simulink model "Lab_1.1_1.3"  (R2025a)
settings: Solver=FixedStepAuto  StartTime=0.0  StopTime=inf  RelTol=1e-3  EnableMultiTasking=on
libraries: fl_lib x18, nesl_utility x18, stm32f4xxblockslib x8, ee_lib x6, dspstat3 x2
settings Model: STM32="{\"AnalogInput\":[{\"ID\":\"test_poten:20\"},{\"ID\":\"test_poten:28\"},{\"ID\":\"ADC_reader:28\"},{\"ID\":\"ADC_reader:20\"},{\"ID\":\"ADC_reader:14\"},{\"ID\":\"ADC_reader:11\"},{\"ID\":\"ADC_reader:8\"},{\"ID\":\"ADC_reader:5\"},{\"ID\":\"ADC_reader:1\"},{\"ID\":\"ADC_reader_simulink:14\"},{\"ID\":\"ADC_reader_simulink:11\"},{\"ID\":\"ADC_reader_simulink:8\"},{\"ID\":\"ADC_reader_simulink:5\"},{\"ID\":\"ADC_reader_simulink:1\"},{\"ID\":\"ADC_reader_simulink:124\"},{\"ID\":\"ADC_reader_simulink:20\"}]}"  Creator=ioonz  LastModifiedBy=Ben
settings OptimizationCC: DefaultParameterBehavior=Inlined  EnhancedBackFolding=on  PassReuseOutputArgsAs=Individual arguments  ZeroExternalMemoryAtStartup=off  ZeroInternalMemoryAtStartup=off  MaxStackSize=512  OptimizeBlockOrder=speed  DifferentSizesBufferReuse=on  OptimizationCustomize=off  EfficientTunableParamExpr=on
settings DebuggingCC: ParameterTunabilityLossMsg=error
settings HardwareCC: ProdBitPerPointer=32.0  ProdBitPerSizeT=32.0  ProdBitPerPtrDiffT=32.0  ProdLargestAtomicInteger=Long  ProdLargestAtomicFloat=Double  ProdWordSize=32.0  ProdLongLongMode=on  ProdHWDeviceType=ARM Compatible->ARM Cortex-M
settings SFSimCC: MATLABDynamicMemAlloc=off
settings RTWCC: SystemTargetFile=ert.tlc  HardwareBoard=STM32G4xx Based  TemplateMakefile=ert_default_tmf  Toolchain=GNU Tools for ARM Embedded Processors  Description=Embedded Coder
settings CodeAppCC: ForceParamTrailComments=on  IgnoreCustomStorageClasses=off  OperatorAnnotations=on  SimulinkDataObjDesc=on  SFDataObjDesc=on  InsertBlockDesc=on
settings ERTTargetCC: ExtModeTransport=3.0  ExtModeStaticAllocSize=2048.0  TargetLangStandard=C99 (ISO)  CodeReplacementLibrary=ARM Cortex-M

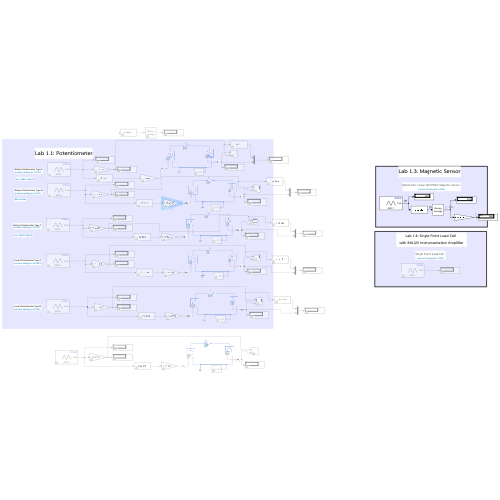
[thumbnail: Simulink's stored preview of the top-level diagram]
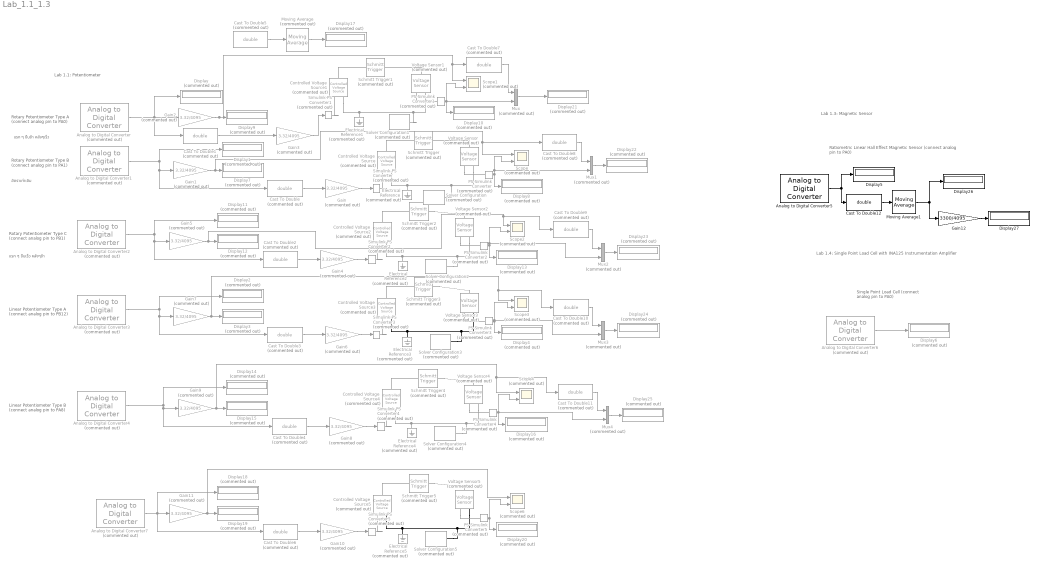
== system Lab_1.1_1.3 ==
  note: Lab 1.1: Potentiometer
  note: Rotary Potentiometer Type A
      | (connect analog pin to PA0)
  note: Rotary Potentiometer Type B
      | (connect analog pin to PA1)
  note: Rotary Potentiometer Type C
      | (connect analog pin to PB1)
  note: Linear Potentiometer Type A
      | (connect analog pin to PB12)
  note: Linear Potentiometer Type B
      | (connect analog pin to PA8)
  note: Ratiometric Linear Hall Effect Magnetic Sensor
      | (connect analog pin to PA0)
  note: Single Point Load Cell
      | (connect analog pin to PA0)
  note: Lab 1.3: Magnetic Sensor
  note: Lab 1.4: Single Point Load Cell
      | with INA125 Instrumentation Amplifier
  note: แรก ๆ ขึ้นเร็ว หลังๆช้า
  note: แรก ๆ ขึ้นช้า หลังๆเร็ว
  note: อัตราเท่าเดิม
  Analog to Digital Converter : stm32f4xxblockslib/Analog to Digital Converter  Commented=on  ADCModule=ADC1  ConversionGroup=Regular  TriggerMode=Trigger and read  NumberOfConversions=1  EnableBufferConv=off  BufferLength=1  OutputStatus=off  SampleTime=-1  EnableSimPort=off  hoistedMaskSrc=ECSoC/ECSimCodegen/Analog to Digital Converter
  Analog to Digital Converter1 : stm32f4xxblockslib/Analog to Digital Converter  Commented=on  ADCModule=ADC2  ConversionGroup=Regular  TriggerMode=Trigger and read  NumberOfConversions=1  EnableBufferConv=off  BufferLength=1  OutputStatus=off  SampleTime=-1  EnableSimPort=off  hoistedMaskSrc=ECSoC/ECSimCodegen/Analog to Digital Converter
  Analog to Digital Converter2 : stm32f4xxblockslib/Analog to Digital Converter  Commented=on  ADCModule=ADC3  ConversionGroup=Regular  TriggerMode=Trigger and read  NumberOfConversions=1  EnableBufferConv=off  BufferLength=1  OutputStatus=off  SampleTime=-1  EnableSimPort=off  hoistedMaskSrc=ECSoC/ECSimCodegen/Analog to Digital Converter
  Analog to Digital Converter3 : stm32f4xxblockslib/Analog to Digital Converter  Commented=on  ADCModule=ADC4  ConversionGroup=Regular  TriggerMode=Trigger and read  NumberOfConversions=1  EnableBufferConv=off  BufferLength=1  OutputStatus=off  SampleTime=-1  EnableSimPort=off  hoistedMaskSrc=ECSoC/ECSimCodegen/Analog to Digital Converter
  Analog to Digital Converter4 : stm32f4xxblockslib/Analog to Digital Converter  Commented=on  ADCModule=ADC5  ConversionGroup=Regular  TriggerMode=Trigger and read  NumberOfConversions=1  EnableBufferConv=off  BufferLength=1  OutputStatus=off  SampleTime=-1  EnableSimPort=off  hoistedMaskSrc=ECSoC/ECSimCodegen/Analog to Digital Converter
  Analog to Digital Converter5 : stm32f4xxblockslib/Analog to Digital Converter  ADCModule=ADC1  ConversionGroup=Regular  TriggerMode=Trigger and read  NumberOfConversions=1  EnableBufferConv=off  BufferLength=1  OutputStatus=off  SampleTime=-1  EnableSimPort=off  hoistedMaskSrc=ECSoC/ECSimCodegen/Analog to Digital Converter
  Analog to Digital Converter6 : stm32f4xxblockslib/Analog to Digital Converter  Commented=on  ADCModule=ADC1  ConversionGroup=Regular  TriggerMode=Trigger and read  NumberOfConversions=1  EnableBufferConv=off  BufferLength=1  OutputStatus=off  SampleTime=-1  EnableSimPort=off  hoistedMaskSrc=ECSoC/ECSimCodegen/Analog to Digital Converter
  Analog to Digital Converter7 : stm32f4xxblockslib/Analog to Digital Converter  Commented=on  ADCModule=ADC5  ConversionGroup=Regular  TriggerMode=Trigger and read  NumberOfConversions=1  EnableBufferConv=off  BufferLength=1  OutputStatus=off  SampleTime=-1  EnableSimPort=off  hoistedMaskSrc=ECSoC/ECSimCodegen/Analog to Digital Converter
  Cast To Double{,1..11} (12 alike) : DataTypeConversion  Commented=on  OutDataTypeStr=double  SaturateOnIntegerOverflow=off  RndMeth=Floor
  Cast To Double12 : DataTypeConversion  OutDataTypeStr=double  SaturateOnIntegerOverflow=off  RndMeth=Floor
  Controlled Voltage Source{,1..5} (6 alike) : fl_lib/Electrical/Electrical Sources/Controlled Voltage Source  Commented=on
  Display{,1..4,6..25} (25 alike) : Display  Commented=on
  Display26 : Display
  Display27 : Display
  Display5 : Display
  Electrical Reference{,1..5} (6 alike) : fl_lib/Electrical/Electrical Elements/Electrical Reference  Commented=on
  Gain{,1..11} (12 alike) : Gain  Commented=on  Gain=3.32/4095
  Gain12 : Gain  Gain=3300/4095
  Moving Average : dspstat3/Moving Average  Commented=on  Method=Sliding window  ForgettingFactorPort=off  SpecifyWindowLength=on  WindowLength=4  OverlapLength=3  AllowArbitraryInputLength=off  ForgettingFactor=0.9  SimulateUsing=Interpreted execution
  Moving Average1 : dspstat3/Moving Average  Method=Sliding window  ForgettingFactorPort=off  SpecifyWindowLength=on  WindowLength=100  OverlapLength=99  AllowArbitraryInputLength=off  ForgettingFactor=0.9  SimulateUsing=Interpreted execution
  Mux{,1..4} (5 alike) : Mux  Commented=on  Inputs=2
  PS-Simulink Converter{,1..5} (6 alike) : nesl_utility/PS-Simulink Converter  Commented=on  PhysicalDomain=network_engine_domain  SubClassName=ps_output  LeftPortType=input  RightPortType=output  PseudoPeriodic=off  Frequencies=[]  VectorFormat=inherit  Unit=inherit  AffineConversion=off
  Schmitt Trigger : ee_lib/Integrated Circuits/Logic/Schmitt Trigger  Commented=on  V_IL=1.1 V  V_IH=1.88 V  C_IN=5 pF  output_type=ee.enum.ic.outputType.linear  V_OL=0 V  V_OH=3 V  V_CC=5 V  V_meas=5 V  R_OUT=25 Ohm  R_OH=[25, 250] Ohm  I_OH=63 mA  R_OL=[30, 800] Ohm  I_OL=-45 mA  Delay=25 ns  Ron=5 Ohm  Vf=0.6 V  output_state=ee.enum.ic.initialState.low
      settings: InternalSimscapePortConfiguration="{\"Bottom\":[],\"Left\":[{\"id\":\"A\",\"label\":\"\",\"type\":\"foundation.electrical.electrical\"}],\"Right\":[{\"id\":\"J\",\"label\":\"\",\"type\":\"foundation.electrical.electrical\"}],\"Top\":[]}"
  Schmitt Trigger1 : ee_lib/Integrated Circuits/Logic/Schmitt Trigger  Commented=on  V_IL=1.5 V  V_IH=2.2 V  C_IN=5 pF  output_type=ee.enum.ic.outputType.linear  V_OL=0 V  V_OH=3 V  V_CC=5 V  V_meas=5 V  R_OUT=25 Ohm  R_OH=[25, 250] Ohm  I_OH=63 mA  R_OL=[30, 800] Ohm  I_OL=-45 mA  Delay=25 ns  Ron=5 Ohm  Vf=0.6 V  output_state=ee.enum.ic.initialState.low
      settings: InternalSimscapePortConfiguration="{\"Bottom\":[],\"Left\":[{\"id\":\"A\",\"label\":\"\",\"type\":\"foundation.electrical.electrical\"}],\"Right\":[{\"id\":\"J\",\"label\":\"\",\"type\":\"foundation.electrical.electrical\"}],\"Top\":[]}"
  Schmitt Trigger2 : ee_lib/Integrated Circuits/Logic/Schmitt Trigger  Commented=on  V_IL=1.147 V  V_IH=1.9 V  C_IN=5 pF  output_type=ee.enum.ic.outputType.linear  V_OL=0 V  V_OH=3 V  V_CC=5 V  V_meas=5 V  R_OUT=25 Ohm  R_OH=[25, 250] Ohm  I_OH=63 mA  R_OL=[30, 800] Ohm  I_OL=-45 mA  Delay=25 ns  Ron=5 Ohm  Vf=0.6 V  output_state=ee.enum.ic.initialState.low
      settings: InternalSimscapePortConfiguration="{\"Bottom\":[],\"Left\":[{\"id\":\"A\",\"label\":\"\",\"type\":\"foundation.electrical.electrical\"}],\"Right\":[{\"id\":\"J\",\"label\":\"\",\"type\":\"foundation.electrical.electrical\"}],\"Top\":[]}"
  Schmitt Trigger3 : ee_lib/Integrated Circuits/Logic/Schmitt Trigger  Commented=on  V_IL=1.22 V  V_IH=1.81 V  C_IN=5 pF  output_type=ee.enum.ic.outputType.linear  V_OL=0 V  V_OH=3 V  V_CC=5 V  V_meas=5 V  R_OUT=25 Ohm  R_OH=[25, 250] Ohm  I_OH=63 mA  R_OL=[30, 800] Ohm  I_OL=-45 mA  Delay=25 ns  Ron=5 Ohm  Vf=0.6 V  output_state=ee.enum.ic.initialState.low
      settings: InternalSimscapePortConfiguration="{\"Bottom\":[],\"Left\":[{\"id\":\"A\",\"label\":\"\",\"type\":\"foundation.electrical.electrical\"}],\"Right\":[{\"id\":\"J\",\"label\":\"\",\"type\":\"foundation.electrical.electrical\"}],\"Top\":[]}"
  Schmitt Trigger4 : ee_lib/Integrated Circuits/Logic/Schmitt Trigger  Commented=on  V_IL=1.52 V  V_IH=2.14 V  C_IN=5 pF  output_type=ee.enum.ic.outputType.linear  V_OL=0 V  V_OH=3 V  V_CC=5 V  V_meas=5 V  R_OUT=25 Ohm  R_OH=[25, 250] Ohm  I_OH=63 mA  R_OL=[30, 800] Ohm  I_OL=-45 mA  Delay=25 ns  Ron=5 Ohm  Vf=0.6 V  output_state=ee.enum.ic.initialState.low
      settings: InternalSimscapePortConfiguration="{\"Bottom\":[],\"Left\":[{\"id\":\"A\",\"label\":\"\",\"type\":\"foundation.electrical.electrical\"}],\"Right\":[{\"id\":\"J\",\"label\":\"\",\"type\":\"foundation.electrical.electrical\"}],\"Top\":[]}"
  Schmitt Trigger5 : ee_lib/Integrated Circuits/Logic/Schmitt Trigger  Commented=on  V_IL=1.1 V  V_IH=2.5 V  C_IN=5 pF  output_type=ee.enum.ic.outputType.linear  V_OL=0 V  V_OH=3 V  V_CC=5 V  V_meas=5 V  R_OUT=25 Ohm  R_OH=[25, 250] Ohm  I_OH=63 mA  R_OL=[30, 800] Ohm  I_OL=-45 mA  Delay=25 ns  Ron=5 Ohm  Vf=0.6 V  output_state=ee.enum.ic.initialState.low
      settings: InternalSimscapePortConfiguration="{\"Bottom\":[],\"Left\":[{\"id\":\"A\",\"label\":\"\",\"type\":\"foundation.electrical.electrical\"}],\"Right\":[{\"id\":\"J\",\"label\":\"\",\"type\":\"foundation.electrical.electrical\"}],\"Top\":[]}"
  Scope{,1..4,6} (6 alike) : Scope  Commented=on  NumInputPorts=2
      Scope settings: ActiveDisplayYMinimum=-0.35294750562766508  ActiveDisplayYMaximum=3.797040042962041
      Scope1 settings: ActiveDisplayYMinimum=-0.58406379051125068  ActiveDisplayYMaximum=3.773423135507942
      Scope2 settings: ActiveDisplayYMinimum=-1.069924034550259  ActiveDisplayYMaximum=5.3680687455364664  DataLoggingVariableName=ScopeData2
      Scope3 settings: ActiveDisplayYMinimum=-0.37499999999999989  ActiveDisplayYMaximum=3.375  DataLoggingVariableName=ScopeData3
      Scope4 settings: ActiveDisplayYMinimum=-1.4986962919239719  ActiveDisplayYMaximum=2.4207253436759375  DataLoggingVariableName=ScopeData4
      Scope6 settings: ActiveDisplayYMinimum=-1.3215835316863527  ActiveDisplayYMaximum=4.9393706253992313  DataLoggingVariableName=ScopeData6
  Simulink-PS Converter{,1..5} (6 alike) : nesl_utility/Simulink-PS Converter  Commented=on  PhysicalDomain=network_engine_domain  SubClassName=ps_input  LeftPortType=input  RightPortType=output  PseudoPeriodic=off  Frequencies=[]  NoiseDistribution=none  NoiseParameters=[]  Unit=1  AffineConversion=off  FilteringAndDerivatives=provide  SimscapeFilterOrder=1  InputFilterTimeConstant=0.001  UdotUserProvided=0
  Solver Configuration{,1..5} (6 alike) : nesl_utility/Solver Configuration  Commented=on  PhysicalDomain=network_engine_domain  SubClassName=solver  LeftPortType=input  RightPortType=generic  Tones=[]  Harmonics=[]  SimulateNoise=off  Profile=off  UseLocalSampling=off  EnableSwitchedLinearOptims=on  FrequencyDomain=off  UseCCode=off  RelTol=0.001  AbsTol=0.001  MinStep=1e-09  ToWorkspace=off  RevertToSquareIcSolve=off  NumHomotopyIterations=100  PhasorMode=off  PhasorModeNumHarmonics=1  ConsistencySolver=NEWTON_XTOL_AFTER_FTOL  IndexReductionMethod=DerivativeReplacement  DoDC=off  ResidualTolerance=1e-09  ConsistencyTolSource=LOCAL  ConsistencyAbsTol=0.001  ConsistencyRelTol=0.001  ConsistencyTolFactor=0.001  UseLocalSolver=on  LocalSolverChoice=NE_BACKWARD_EULER_ADVANCER  ResolveIndetEquations=on  FunctionEvalNumThread=1  LocalSolverSampleTime=0.001  DoFixedCost=off  MaxNonlinIter=3  MaxModeIter=2  ComputeImpulses=off  ImpulseIterations=2  LinearAlgebra=auto  LinearAlgebraNumThread=0  EquationFormulation=NE_TIME_EF  DelaysMemoryBudget=1024  AutomaticFiltering=on  FilteringTimeConstant=0.001  PartitionStorageMethod=AS_NEEDED  PartitionMemoryBudget=1024  PartitionMethod=ROBUST  MultibodyUseLocalSolver=on  MultibodyLocalSolverChoice=ODE1  MultibodyLocalSolverSampleTime=0.001
  Voltage Sensor{,1..5} (6 alike) : fl_lib/Electrical/Electrical Sensors/Voltage Sensor  Commented=on
  wires:
  Analog to Digital Converter/1 -> Cast To Double1/1, Gain2/1, Display/1
  Analog to Digital Converter5/1 -> Cast To Double12/1, Display5/1
  Analog to Digital Converter6/1 -> Display6/1
  Gain/1 -> Simulink-PS Converter/1
  Analog to Digital Converter1/1 -> Cast To Double/1, Gain1/1, Display1/1
  Cast To Double/1 -> Gain/1
  Gain1/1 -> Cast To Double8/1, Scope/1, Display7/1
  Gain2/1 -> Scope1/1, Cast To Double7/1, Display9/1
  Cast To Double1/1 -> Gain3/1
  PS-Simulink Converter1/1 -> Mux/2, Display10/1, Scope1/2
  Gain3/1 -> Simulink-PS Converter1/1
  Gain5/1 -> Cast To Double9/1, Scope2/1, Display12/1
  Cast To Double2/1 -> Gain4/1
  Analog to Digital Converter2/1 -> Display11/1, Gain5/1, Cast To Double2/1
  Gain4/1 -> Simulink-PS Converter2/1
  Gain6/1 -> Simulink-PS Converter3/1
  Analog to Digital Converter3/1 -> Cast To Double3/1, Gain7/1, Display2/1
  Cast To Double3/1 -> Gain6/1
  Gain7/1 -> Scope3/1, Cast To Double10/1, Display3/1
  PS-Simulink Converter4/1 -> Mux4/2, Display16/1, Scope4/2
  Gain9/1 -> Cast To Double11/1, Scope4/1, Display15/1
  Cast To Double4/1 -> Gain8/1
  Analog to Digital Converter4/1 -> Display14/1, Gain9/1, Cast To Double4/1
  Gain8/1 -> Simulink-PS Converter4/1
  PS-Simulink Converter2/1 -> Mux2/2, Scope2/2, Display13/1
  PS-Simulink Converter/1 -> Mux1/2, Scope/2, Display8/1
  PS-Simulink Converter3/1 -> Mux3/2, Scope3/2, Display4/1
  Cast To Double5/1 -> Moving Average/1
  Moving Average/1 -> Display17/1
  Gain10/1 -> Simulink-PS Converter5/1
  Analog to Digital Converter7/1 -> Gain11/1, Display18/1, Cast To Double6/1
  Cast To Double6/1 -> Gain10/1
  Gain11/1 -> Display19/1, Scope6/1
  PS-Simulink Converter5/1 -> Scope6/2, Display20/1
  Mux/1 -> Display21/1
  Cast To Double7/1 -> Mux/1
  Cast To Double8/1 -> Mux1/1
  Mux1/1 -> Display22/1
  Mux2/1 -> Display23/1
  Cast To Double9/1 -> Mux2/1
  Cast To Double10/1 -> Mux3/1
  Mux3/1 -> Display24/1
  Mux4/1 -> Display25/1
  Cast To Double11/1 -> Mux4/1
  Cast To Double12/1 -> Moving Average1/1
  Moving Average1/1 -> Display26/1, Gain12/1
  Gain12/1 -> Display27/1
  connections:
  Simulink-PS Converter/RConn1 -- Controlled Voltage Source/RConn1
  Controlled Voltage Source/RConn2 -- Solver Configuration/RConn1 -- Voltage Sensor/RConn2 -- Electrical Reference/LConn1
  Controlled Voltage Source/LConn1 -- Schmitt Trigger/LConn1
  Voltage Sensor/LConn1 -- Schmitt Trigger/RConn1
  Voltage Sensor/RConn1 -- PS-Simulink Converter/LConn1
  Solver Configuration1/RConn1 -- Voltage Sensor1/RConn2 -- Controlled Voltage Source1/RConn2 -- Electrical Reference1/LConn1
  Voltage Sensor1/RConn1 -- PS-Simulink Converter1/LConn1
  Controlled Voltage Source1/LConn1 -- Schmitt Trigger1/LConn1
  Simulink-PS Converter1/RConn1 -- Controlled Voltage Source1/RConn1
  Voltage Sensor1/LConn1 -- Schmitt Trigger1/RConn1
  Solver Configuration2/RConn1 -- Electrical Reference2/LConn1 -- Controlled Voltage Source2/RConn2 -- Voltage Sensor2/RConn2
  Voltage Sensor2/RConn1 -- PS-Simulink Converter2/LConn1
  Simulink-PS Converter2/RConn1 -- Controlled Voltage Source2/RConn1
  Controlled Voltage Source2/LConn1 -- Schmitt Trigger2/LConn1
  Schmitt Trigger2/RConn1 -- Voltage Sensor2/LConn1
  Electrical Reference3/LConn1 -- Solver Configuration3/RConn1 -- Voltage Sensor3/RConn2 -- Controlled Voltage Source3/RConn2
  Controlled Voltage Source3/LConn1 -- Schmitt Trigger3/LConn1
  Simulink-PS Converter3/RConn1 -- Controlled Voltage Source3/RConn1
  Schmitt Trigger3/RConn1 -- Voltage Sensor3/LConn1
  Voltage Sensor3/RConn1 -- PS-Simulink Converter3/LConn1
  Solver Configuration4/RConn1 -- Electrical Reference4/LConn1 -- Controlled Voltage Source4/RConn2 -- Voltage Sensor4/RConn2
  Schmitt Trigger4/RConn1 -- Voltage Sensor4/LConn1
  Simulink-PS Converter4/RConn1 -- Controlled Voltage Source4/RConn1
  Voltage Sensor4/RConn1 -- PS-Simulink Converter4/LConn1
  Controlled Voltage Source4/LConn1 -- Schmitt Trigger4/LConn1
  Electrical Reference5/LConn1 -- Solver Configuration5/RConn1 -- Voltage Sensor5/RConn2 -- Controlled Voltage Source5/RConn2
  Voltage Sensor5/RConn1 -- PS-Simulink Converter5/LConn1
  Simulink-PS Converter5/RConn1 -- Controlled Voltage Source5/RConn1
  Schmitt Trigger5/RConn1 -- Voltage Sensor5/LConn1
  Controlled Voltage Source5/LConn1 -- Schmitt Trigger5/LConn1
